simulink subsystem "PvtSubSys_LATC"  (R2020b)
settings: Solver=VariableStepAuto  StartTime=0.0  StopTime=10.0  RelTol=1e-3
undefined symbols (not defined in the file or in its folder): LCS_PLAN_PreViewIdxNum, LCS_PLAN_PreViewIdxSW_b, P_Global_CharSpd_ms, P_Global_SteeringAngleRatio, P_Global_WheelBase_m, P_LCS_DetNoOverRide_DrvTrq_TH, P_LCS_DetOverRide_DrvTrq_TH, P_LCS_ESS_AngleSlope_Limit, P_LCS_ESS_LogicTest_Enable, P_LCS_ESS_NotActiveFlgDelayTime, P_LCS_ESS_NotActiveFlgDelayTimeSW, P_LCS_ESS_SteerAngleErr, P_LCS_ESS_SteerAngleFilterTime, P_LCS_ESS_TarAngleFilterTime, P_LCS_ESSAngleSW, P_LCS_ESSOverrideTime1, P_LCS_ESSOverrideTime2, P_LCS_ESSOverrideTime3, P_LCS_ESSOverrideValue1, P_LCS_ESSOverrideValue2, P_LCS_IN_Offset_Test_SW, P_LCS_IN_Offset_Test_Value, P_LCS_LATC_AngleFilterTime_s, P_LCS_LATC_CurOffsetA2FliterT_s, P_LCS_LATC_CurOffsetCurve_TabX_m, P_LCS_LATC_CurOffsetCurveFliterTime_Tab_s, P_LCS_LATC_CurOffsetVehicleSpdLimitValue_degs, P_LCS_LATC_DeltaEps_Tab_s, P_LCS_LATC_DxOffset_Sw, P_LCS_LATC_ELKAngleSlope_ratio, P_LCS_LATC_ELKMaxLatAcc_ms2, P_LCS_LATC_ESSA0Dis_TabX_m, P_LCS_LATC_ESSAddAngleSlope_Tab_degs, P_LCS_LATC_ESSAESAngleSlope_Tab_degs, P_LCS_LATC_ESSAngleSlope_ratio, P_LCS_LATC_ESSMaxLatAcc_ms2, P_LCS_LATC_LCAngleSlope_ratio, P_LCS_LATC_LCAngleSlope_Tab_degs, P_LCS_LATC_LCCancleMaxLatAcc_ms2, P_LCS_LATC_LCEcoAngleSlope_ratio, P_LCS_LATC_LCEcoAngleSlope_Tab_degs, P_LCS_LATC_LCEcoMaxLatAcc_ms2, P_LCS_LATC_LCKAngleSlope_ratio, P_LCS_LATC_LCKAngleSlope_Tab_degs, P_LCS_LATC_LCKIEAngleSlope_ratio, P_LCS_LATC_LCKIEAngleSlope_Tab_degs, P_LCS_LATC_LCKIEMaxLatAcc_ms2, P_LCS_LATC_LCKMaxLatAcc_ms2, P_LCS_LATC_LCNormalAngleSlope_ratio, P_LCS_LATC_LCNormalAngleSlope_Tab_degs, P_LCS_LATC_LCNormalMaxLatAcc_ms2, P_LCS_LATC_LCSportAngleSlope_ratio, P_LCS_LATC_LCSportAngleSlope_Tab_degs, P_LCS_LATC_LCSportMaxLatAcc_ms2, P_LCS_LATC_LKAAngleSlope_ratio, P_LCS_LATC_LKAAngleSlope_Tab_degs, P_LCS_LATC_LKAMaxLatAcc_ms2, P_LCS_LATC_MatrixQ1_st, P_LCS_LATC_MatrixQ3_st, P_LCS_LATC_MatrixR_st ... (+71)
libraries: simulink x38
(part 3 of 6)

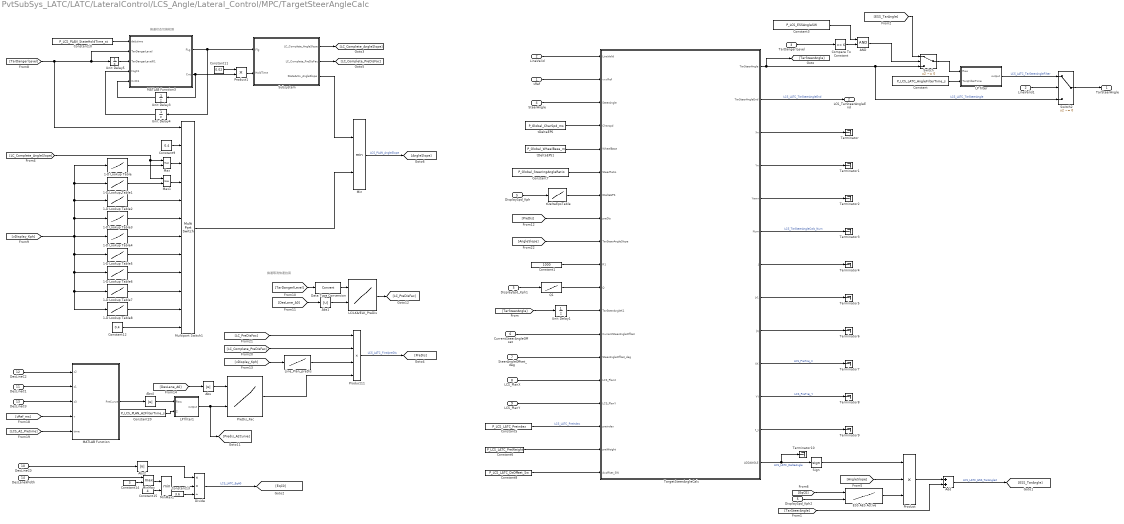
== system PvtSubSys_LATC/LATC/LateralControl/LCS_Angle/Lateral_Control/MPC/TargetSteerAngleCalc ==
  note: 换道状态切换检测
  note: 换道取消快速拉回
  vRef : Inport
  LineValid : Inport  Port=2
  TarDangerlLevel : Inport  Port=3
  SteerAngle : Inport  Port=4
  DisplaySpd_Kph : Inport  Port=5
  CurrentSteerAngleOffset : Inport  Port=6
  SteerAngleOffset_deg : Inport  Port=7
  LCS_PlanX : Inport  Port=8
  LCS_PlanY : Inport  Port=9
  DesLineC0 : Inport  Port=10
  DesLineC1 : Inport  Port=11
  DesLineC2 : Inport  Port=12
  DesLineC3 : Inport  Port=13
  DesLaneWidth : Inport  Port=14
  1-D Lookup Table : Lookup_n-D  NumberOfTableDimensions=1  BreakpointsForDimension1=P_LCS_LATC_VehicleSpd_TabX_Kph  Table=P_LCS_LATC_LCKAngleSlope_Tab_degs  InternalRulePriority=Speed  RndMeth=Simplest  InputSameDT=on
  1-D Lookup Table1 : Lookup_n-D  NumberOfTableDimensions=1  BreakpointsForDimension1=P_LCS_LATC_VehicleSpd_TabX_Kph  Table=P_LCS_LATC_LCKIEAngleSlope_Tab_degs  InternalRulePriority=Speed  RndMeth=Simplest  InputSameDT=on
  1-D Lookup Table2 : Lookup_n-D  NumberOfTableDimensions=1  BreakpointsForDimension1=P_LCS_LATC_VehicleSpd_TabX_Kph  Table=P_LCS_LATC_LCNormalAngleSlope_Tab_degs  InternalRulePriority=Speed  RndMeth=Simplest  InputSameDT=on
  1-D Lookup Table3 : Lookup_n-D  NumberOfTableDimensions=1  BreakpointsForDimension1=P_LCS_LATC_VehicleSpd_TabX_Kph  Table=P_LCS_LATC_LKAAngleSlope_Tab_degs  InternalRulePriority=Speed  RndMeth=Simplest  InputSameDT=on
  1-D Lookup Table4 : Lookup_n-D  NumberOfTableDimensions=1  BreakpointsForDimension1=P_LCS_LATC_VehicleSpd_TabX_Kph  Table=P_LCS_PLAN_ELKAngleSlope_Tab_degs  InternalRulePriority=Speed  RndMeth=Simplest  InputSameDT=on
  1-D Lookup Table5 : Lookup_n-D  NumberOfTableDimensions=1  BreakpointsForDimension1=P_LCS_LATC_VehicleSpd_TabX_Kph  Table=P_LCS_LATC_ESSAESAngleSlope_Tab_degs  InternalRulePriority=Speed  RndMeth=Simplest  InputSameDT=on
  1-D Lookup Table6 : Lookup_n-D  NumberOfTableDimensions=1  BreakpointsForDimension1=P_LCS_LATC_VehicleSpd_TabX_Kph  Table=P_LCS_LATC_LCEcoAngleSlope_Tab_degs  InternalRulePriority=Speed  RndMeth=Simplest  InputSameDT=on
  1-D Lookup Table7 : Lookup_n-D  NumberOfTableDimensions=1  BreakpointsForDimension1=P_LCS_LATC_VehicleSpd_TabX_Kph  Table=P_LCS_LATC_LCSportAngleSlope_Tab_degs  InternalRulePriority=Speed  RndMeth=Simplest  InputSameDT=on
  1-D Lookup Table8 : Lookup_n-D  NumberOfTableDimensions=1  BreakpointsForDimension1=P_LCS_LATC_VehicleSpd_TabX_Kph  Table=P_LCS_LATC_LCAngleSlope_Tab_degs  InternalRulePriority=Speed  RndMeth=Simplest  InputSameDT=on
  AND : Logic  AllPortsSameDT=off  OutDataTypeStr=boolean
  Abs{,1..2,4} (4 alike) : Abs
  Add : Sum
  Compare To Constant : simulink/Logic and Bit Operations/Compare To Constant  relop===  const=6  OutDataTypeStr=boolean
  Constant : Constant  Value=P_LCS_LATC_AngleFilterTime_s  OutDataTypeStr=single
  Constant1 : Constant  Value=1000  OutDataTypeStr=single
  Constant10 : Constant  Value=P_LCS_PLAN_StateHoldTime_st  OutDataTypeStr=uint16
  Constant11 : Constant  Value=0.02
  Constant12 : Constant  Value=0.4  OutDataTypeStr=single
  Constant13 : Constant  Value=3.6  OutDataTypeStr=single
  Constant14 : Constant  Value=3  OutDataTypeStr=single
  Constant15 : Constant  Value=4  OutDataTypeStr=single
  Constant20 : Constant  Value=P_LCS_PLAN_A2FliterTime_s
  Constant3 : Constant  Value=P_LCS_ESSAngleSW  OutDataTypeStr=boolean
  Constant5 : Constant  Value=P_LCS_LATC_Preindex  OutDataTypeStr=single
  Constant6 : Constant  Value=P_LCS_LATC_PreWeight  OutDataTypeStr=single
  Constant7 : Constant  Value=P_Global_SteeringAngleRatio  OutDataTypeStr=single
  Constant8 : Constant  Value=P_LCS_LATC_DxOffset_Sw
  Constant9 : Constant  Value=0.4  OutDataTypeStr=single
  Data Type Conversion : DataTypeConversion
  DisplaySpd_Kph1 : InportShadow  Port=5
  DisplaySpd_Kph2 : InportShadow  Port=5
  Divide : Product  Inputs=**/
  ESS AES Active : Lookup_n-D  BreakpointsForDimension1=P_LCS_LATC_ESSA0Dis_TabX_m  BreakpointsForDimension2=P_LCS_LATC_VehicleSpd_TabX_Kph  Table=P_LCS_LATC_ESSAddAngleSlope_Tab_degs  ExtrapMethod=Clip  UseLastTableValue=on  InternalRulePriority=Speed  OutDataTypeStr=single  RndMeth=Simplest
      settings: InputPortMap=u0,u1
  LC/LKA/ELK_PreDis : Lookup_n-D  BreakpointsForDimension1=P_LCS_PLAN_TarDangerlLevel_Tabx_st  BreakpointsForDimension2=P_LCS_PLAN_DesLineA0_TabY_m  Table=P_LCS_PLAN_LCPreDisFac_ratio  ExtrapMethod=Clip  UseLastTableValue=on  InternalRulePriority=Speed  RndMeth=Simplest  InputSameDT=on
      settings: InputPortMap=u0,u1
  LP filter : Subsystem
  LP filter1 : Subsystem
  LineValid1 : InportShadow  Port=2
  Line_Plan_preDis : Lookup_n-D  NumberOfTableDimensions=1  BreakpointsForDimension1=P_LCS_PLAN_VehicleSpd_TabX_Kph  Table=P_LCS_PLAN_PreDis_Tab_m  ExtrapMethod=Clip  UseLastTableValue=on  InternalRulePriority=Speed  RndMeth=Simplest  InputSameDT=on
  MATLAB Function : MATLAB Function  TreatAsAtomicUnit=on
  MATLAB Function3 : MATLAB Function  TreatAsAtomicUnit=on
  Max : MinMax  Function=max  Inputs=2
  Max1 : MinMax  Function=max  Inputs=2
  Min : MinMax  Inputs=2
  MinMax : MinMax  Function=max  Inputs=2
  MinMax1 : MinMax  Inputs=2
  Multiport Switch1 : MultiPortSwitch  DataPortOrder=Zero-based contiguous  Inputs=11  zeroidx=on
  PreDis_Fac : Lookup_n-D  BreakpointsForDimension1=P_LCS_PLAN_DesLineA0_TabX_m  BreakpointsForDimension2=P_LCS_PLAN_PreDisCurve_TabY_m  Table=P_LCS_PlLAN_PreDisFac_Tab_ratio  ExtrapMethod=Clip  UseLastTableValue=on  InternalRulePriority=Speed  RndMeth=Simplest  InputSameDT=on
      settings: InputPortMap=u0,u1
  Product : Product  Inputs=3  OutDataTypeStr=single
  Product1 : Product
  Product11 : Product  Inputs=4
  Q1 : Lookup_n-D  NumberOfTableDimensions=1  BreakpointsForDimension1=[0,5,10,15,20,25,30,35,40,60,80,90,100,110,120,140]  Table=[0,0,0,0,0,0,0,0,0,0,0,0,0,0,0,0]  InternalRulePriority=Speed  RndMeth=Simplest  InputSameDT=on
  Sign : Signum
  Subsystem : Subsystem
  Switch : Switch  Criteria=u2 ~= 0
  Switch2 : Switch  Criteria=u2 ~= 0
  TargetSteerAngleCalc : MATLAB Function  TreatAsAtomicUnit=on
  Terminator{,1..10} (11 alike) : Terminator
  Unit Delay{1,3..5} (4 alike) : UnitDelay  SampleTime=-1  HasFrameUpgradeWarning=on
  tDeltaEPS : Constant  Value=P_Global_CharSpd_ms
  tDeltaEPS1 : Constant  Value=P_Global_WheelBase_m
  tDeltaEpsTable : Lookup_n-D  NumberOfTableDimensions=1  BreakpointsForDimension1=P_LCS_PLAN_VehicleSpd_TabX_Kph  Table=P_LCS_LATC_DeltaEps_Tab_s  ExtrapMethod=Clip  InternalRulePriority=Speed  RndMeth=Simplest  InputSameDT=on
  TarSteerAngle : Outport
  LCS_TarSteerAngleEnd : Outport  Port=2
  wires:
  Constant8/1 -> TargetSteerAngleCalc/19(dxoffset_SW)
  Constant6/1 -> TargetSteerAngleCalc/18(preWeight)
  Constant5/1 -> TargetSteerAngleCalc/17(preindex)  "LCS_LATC_PreIndex"
  LCS_PlanY/1 -> TargetSteerAngleCalc/16(LCS_PlanY)
  LCS_PlanX/1 -> TargetSteerAngleCalc/15(LCS_PlanX)
  LineValid1/1 -> Switch2/2
  ESS AES Active/1 -> Product/3
  DisplaySpd_Kph2/1 -> ESS AES Active/2
  [EqC0] -> ESS AES Active/1
  TarDangerlLevel/1 -> Compare To Constant/1
  TargetSteerAngleCalc/13(ADDANGLE) -> Sign/1, Terminator10/1  "LCS_LATC_DeltaAngle"
  Sign/1 -> Product/1
  [AngleSlope] -> Product/2
  Product/1 -> Add/1
  [TarSteerAngle] -> Add/2
  Add/1 -> [ESS_TarAngle]  "LCS_LATC_ESS_TarAngle2"
  TargetSteerAngleCalc/1(TarSteerAngle) -> Switch/3, Switch2/3, [TarSteerAngle]  "LCS_LATC_TarSteerAngle"
  Constant/1 -> LP filter/2(TorqFilterTime)
  LP filter/1(output) -> Switch2/1  "LCS_LATC_TarSteerAngleFilter"
  Switch/1 -> LP filter/1(Raw)
  [ESS_TarAngle] -> Switch/1
  Constant3/1 -> AND/1
  Compare To Constant/1 -> AND/2
  AND/1 -> Switch/2
  Switch2/1 -> TarSteerAngle/1
  TargetSteerAngleCalc/12(t_y) -> Terminator9/1
  TargetSteerAngleCalc/2(TarSteerAngleEnd) -> LCS_TarSteerAngleEnd/1  "LCS_LATC_TarSteerAngleEnd"
  [PreDis] -> TargetSteerAngleCalc/8(preDis)
  [AngleSlope] -> TargetSteerAngleCalc/9(TarSteerAngleSlope)
  SteerAngle/1 -> TargetSteerAngleCalc/3(SteerAngle)
  vRef/1 -> TargetSteerAngleCalc/2(vxvRef)
  TargetSteerAngleCalc/11(YY) -> Terminator8/1  "LCS_PreTraj_Y"
  TargetSteerAngleCalc/10(XX) -> Terminator7/1  "LCS_PreTraj_X"
  Constant1/1 -> TargetSteerAngleCalc/10(R1)
  TargetSteerAngleCalc/9(Jq) -> Terminator6/1
  TargetSteerAngleCalc/8(Jr1) -> Terminator5/1
  TargetSteerAngleCalc/7(J) -> Terminator4/1
  TargetSteerAngleCalc/6(Num) -> Terminator3/1  "LCS_TarSteerAngleCalc_Num"
  TargetSteerAngleCalc/5(Yawn) -> Terminator2/1
  TargetSteerAngleCalc/4(Yn) -> Terminator1/1
  TargetSteerAngleCalc/3(Xn) -> Terminator/1
  Constant7/1 -> TargetSteerAngleCalc/6(SteerRatio)
  tDeltaEpsTable/1 -> TargetSteerAngleCalc/7(tDeltaEPS)
  DisplaySpd_Kph/1 -> tDeltaEpsTable/1
  tDeltaEPS/1 -> TargetSteerAngleCalc/4(Charspd)
  tDeltaEPS1/1 -> TargetSteerAngleCalc/5(WheelBase)
  [TarSteerAngle] -> Unit Delay1/1
  Unit Delay1/1 -> TargetSteerAngleCalc/12(TarSteerAngleK1)
  Q1/1 -> TargetSteerAngleCalc/11(Q)
  DisplaySpd_Kph1/1 -> Q1/1
  CurrentSteerAngleOffset/1 -> TargetSteerAngleCalc/13(CurrentSteerAngleOffset)
  LineValid/1 -> TargetSteerAngleCalc/1(LineValid)
  SteerAngleOffset_deg/1 -> TargetSteerAngleCalc/14(SteerAngleOffset_deg)
  Constant12/1 -> Multiport Switch1/12
  1-D Lookup Table7/1 -> Multiport Switch1/10
  MATLAB Function3/1(FLg) -> Unit Delay4/1, Subsystem/1(Flg)
  MATLAB Function3/2(Cnt) -> Product1/2, Unit Delay3/1
  Unit Delay3/1 -> MATLAB Function3/5(CntK1)
  1-D Lookup Table4/1 -> Multiport Switch1/7
  1-D Lookup Table/1 -> Max/2
  Unit Delay5/1 -> MATLAB Function3/3(TarDangerLevelK1)
  1-D Lookup Table2/1 -> Multiport Switch1/5
  1-D Lookup Table5/1 -> Multiport Switch1/8
  1-D Lookup Table6/1 -> Multiport Switch1/9
  Max1/1 -> Multiport Switch1/4
  Max/1 -> Multiport Switch1/3
  [LC_Complete_AngleSlope] -> Max1/1, Max/1
  [TarDangerlLevel] -> MATLAB Function3/2(TarDangerLevel), Unit Delay5/1, Multiport Switch1/1
  Constant9/1 -> Multiport Switch1/2
  Constant10/1 -> MATLAB Function3/1(delytime)
  1-D Lookup Table3/1 -> Multiport Switch1/6
  Product1/1 -> Subsystem/2(HoldTime)
  1-D Lookup Table8/1 -> Multiport Switch1/11
  Min/1 -> [AngleSlope]  "LCS_PLAN_AngleSlope"
  Unit Delay4/1 -> MATLAB Function3/4(FLgK1)
  Multiport Switch1/1 -> Min/2
  1-D Lookup Table1/1 -> Max1/2
  Constant11/1 -> Product1/1
  PreDis_Fac/1 -> Product11/4
  Line_Plan_preDis/1 -> Product11/3
  MATLAB Function/1(PreCurve) -> Abs4/1
  DesLineC2/1 -> MATLAB Function/1(c2)
  [vRef_ms] -> MATLAB Function/4(v)
  Data Type Conversion/1 -> LC/LKA/ELK_PreDis/1
  Abs/1 -> PreDis_Fac/1
  [DesLane_A0] -> Abs1/1
  Abs1/1 -> LC/LKA/ELK_PreDis/2
  [vDisplay_Kph] -> Line_Plan_preDis/1
  LC/LKA/ELK_PreDis/1 -> [LC_PreDisFac]
  [TarDangerlLevel] -> Data Type Conversion/1
  [DesLane_A0] -> Abs/1
  DesLineC3/1 -> MATLAB Function/3(c3)
  Constant20/1 -> LP filter1/2(TorqFilterTime)
  Abs4/1 -> LP filter1/1(Raw)
  Product11/1 -> [PreDis]  "LCS_LATC_FinalpreDis"
  [LC_PreDisFac] -> Product11/1
  LP filter1/1(output) -> PreDis_Fac/2, [Predis_A2Curve]
  [LC_Complete_PreDisFac] -> Product11/2
  [LCS_A2_Pretime] -> MATLAB Function/5(time)
  DesLineC1/1 -> MATLAB Function/2(c1)
  [vDisplay_Kph] -> 1-D Lookup Table8/1, 1-D Lookup Table7/1, 1-D Lookup Table6/1, 1-D Lookup Table5/1, 1-D Lookup Table2/1, 1-D Lookup Table1/1, 1-D Lookup Table/1, 1-D Lookup Table3/1, 1-D Lookup Table4/1
  Subsystem/1(LC_Complete_AngleSlope) -> [LC_Complete_AngleSlope]
  Subsystem/3(StateActiv_AngleSlope) -> Min/1
  Subsystem/2(LC_Complete_PreDisFac) -> [LC_Complete_PreDisFac]
  Constant15/1 -> MinMax1/2
  Constant13/1 -> Divide/3
  MinMax1/1 -> Divide/2
  DesLineC0/1 -> Abs2/1
  MinMax/1 -> MinMax1/1
  Divide/1 -> [EqC0]  "LCS_LATC_EqA0"
  Constant14/1 -> MinMax/2
  DesLaneWidth/1 -> MinMax/1
  Abs2/1 -> Divide/1

== system PvtSubSys_LATC/LATC/LateralControl/LCS_Angle/Lateral_Control/MPC/Understeer_Offset_Calc ==
  note: %% 匀速
  SteerAngle_deg : Inport
  PsiDtOpt : Inport  Port=2
  axvRef : Inport  Port=3
  DesLineC2 : Inport  Port=4
  vxvRef : Inport  Port=5
  Abs : Abs
  Abs2 : Abs
  Compare To Constant1 : simulink/Logic and Bit Operations/Compare To Constant  relop=>  const=P_LCS_LATC_CurOffsetVehicleSpdLimitValue_degs  OutDataTypeStr=boolean
  Compare To Constant6 : simulink/Logic and Bit Operations/Compare To Constant  relop=<=  const=1.5  OutDataTypeStr=boolean
  Constant1 : Constant  Value=P_Global_SteeringAngleRatio
  Constant2 : Constant  Value=P_LCS_LATC_CurOffsetA2FliterT_s  OutDataTypeStr=single
  Constant4 : Constant  Value=P_Global_CharSpd_ms
  Constant5 : Constant  Value=P_Global_WheelBase_m
  Constant6 : Constant  Value=57.3  OutDataTypeStr=single
  Enabled Subsystem : Subsystem  TreatAsAtomicUnit=on
  FilterTime2 : Product  Inputs=*//  RndMeth=Zero
  Gain : Gain  Gain=2
  LP filter : Subsystem
  Logical Operator : Logic  AllPortsSameDT=off  OutDataTypeStr=boolean
  Memory52 : Memory  InheritSampleTime=on
  Sum : Sum  Inputs=+-
  Terminator : Terminator
  YOD_Ackman : MATLAB Function  TreatAsAtomicUnit=on
  SteerAngleOffset_deg : Outport
  wires:
  Constant2/1 -> LP filter/2(TorqFilterTime)
  DesLineC2/1 -> Gain/1
  Gain/1 -> Abs/1
  Abs/1 -> LP filter/1(Raw)
  SteerAngle_deg/1 -> FilterTime2/1
  Compare To Constant1/1 -> Logical Operator/2
  YOD_Ackman/2(PsiDtAck) -> Memory52/1, Sum/1
  Enabled Subsystem/1(SteerAngleOffset_deg) -> SteerAngleOffset_deg/1
  Constant5/1 -> YOD_Ackman/3(WheelBase)
  Constant4/1 -> YOD_Ackman/2(Vch)
  Memory52/1 -> YOD_Ackman/5(PsiDtAckK1)
  PsiDtOpt/1 -> Sum/2
  vxvRef/1 -> YOD_Ackman/1(VxvRef), Compare To Constant1/1
  Sum/1 -> Enabled Subsystem/2(Raw)
  Logical Operator/1 -> Enabled Subsystem/Enable, Terminator/1  "LCS_OffSetUpdate_Flg"
  Constant1/1 -> FilterTime2/2
  Constant6/1 -> FilterTime2/3
  YOD_Ackman/1(AckConst) -> Enabled Subsystem/1(AckConst)
  FilterTime2/1 -> YOD_Ackman/4(AlpWheelAngle)
  axvRef/1 -> Abs2/1
  Abs2/1 -> Compare To Constant6/1
  Compare To Constant6/1 -> Logical Operator/1
  LP filter/1(output) -> Enabled Subsystem/3(Curve)

== system PvtSubSys_LATC/LATC/LateralControl/LCS_Angle/Lateral_Control/Trajectory_MPC/Median_Filter ==
  In : Inport
  Constant11 : Constant  Value=P_LCS_LCC_TarAngleFliterWindowSize - single(2)  OutDataTypeStr=single
  Divide1 : Product  Inputs=*/
  Max of Elements1 : MinMax  Function=max
  MinMax2 : MinMax
  Minus1 : Sum  Inputs=--+
  Sum of Elements1 : Sum  Inputs=+
  Tapped Delay1 : simulink/Discrete/Tapped Delay  vinit=0.0  samptime=-1  NumDelays=P_LCS_LCC_TarAngleFliterWindowSize-1  DelayOrder=Newest  includeCurrent=on
  Out : Outport
  wires:
  Max of Elements1/1 -> Minus1/2
  Divide1/1 -> Out/1
  Minus1/1 -> Divide1/1
  In/1 -> Tapped Delay1/1
  MinMax2/1 -> Minus1/1
  Sum of Elements1/1 -> Minus1/3
  Tapped Delay1/1 -> Max of Elements1/1, MinMax2/1, Sum of Elements1/1
  Constant11/1 -> Divide1/2

== system PvtSubSys_LATC/LATC/LateralControl/LCS_Angle/Lateral_Control/Trajectory_MPC/Subsystem5 ==
  raw : Inport
  Slope : Inport  Port=2
  Add : Sum
  Add1 : Sum  Inputs=+-
  Max : MinMax  Inputs=2
  Min : MinMax  Function=max  Inputs=2
  Unit Delay : UnitDelay  InitialCondition=single(0)  SampleTime=-1  HasFrameUpgradeWarning=on
  out : Outport
  wires:
  raw/1 -> Max/2
  Add1/1 -> Min/2
  Add/1 -> Max/1
  Max/1 -> Min/1
  Min/1 -> Unit Delay/1, out/1
  Unit Delay/1 -> Add/1, Add1/1
  Slope/1 -> Add/2, Add1/2

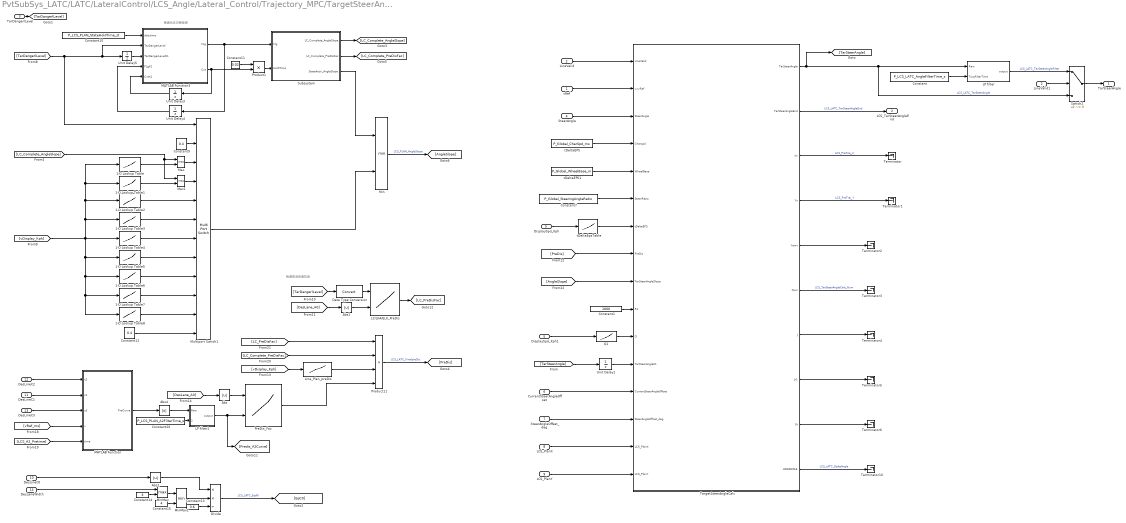
== system PvtSubSys_LATC/LATC/LateralControl/LCS_Angle/Lateral_Control/Trajectory_MPC/TargetSteerAngleCalc ==
  note: 换道取消快速拉回
  note: 换道状态切换检测
  vRef : Inport
  LineValid : Inport  Port=2
  TarDangerlLevel : Inport  Port=3
  SteerAngle : Inport  Port=4
  DisplaySpd_Kph : Inport  Port=5
  CurrentSteerAngleOffset : Inport  Port=6
  SteerAngleOffset_deg : Inport  Port=7
  LCS_PlanX : Inport  Port=8
  LCS_PlanY : Inport  Port=9
  DesLineC0 : Inport  Port=10
  DesLineC1 : Inport  Port=11
  DesLineC2 : Inport  Port=12
  DesLineC3 : Inport  Port=13
  DesLaneWidth : Inport  Port=14
  1-D Lookup Table : Lookup_n-D  NumberOfTableDimensions=1  BreakpointsForDimension1=P_LCS_LATC_VehicleSpd_TabX_Kph  Table=P_LCS_LATC_LCKAngleSlope_Tab_degs  InternalRulePriority=Speed  RndMeth=Simplest  InputSameDT=on
  1-D Lookup Table1 : Lookup_n-D  NumberOfTableDimensions=1  BreakpointsForDimension1=P_LCS_LATC_VehicleSpd_TabX_Kph  Table=P_LCS_LATC_LCKIEAngleSlope_Tab_degs  InternalRulePriority=Speed  RndMeth=Simplest  InputSameDT=on
  1-D Lookup Table2 : Lookup_n-D  NumberOfTableDimensions=1  BreakpointsForDimension1=P_LCS_LATC_VehicleSpd_TabX_Kph  Table=P_LCS_LATC_LCNormalAngleSlope_Tab_degs  InternalRulePriority=Speed  RndMeth=Simplest  InputSameDT=on
  1-D Lookup Table3 : Lookup_n-D  NumberOfTableDimensions=1  BreakpointsForDimension1=P_LCS_LATC_VehicleSpd_TabX_Kph  Table=P_LCS_LATC_LKAAngleSlope_Tab_degs  InternalRulePriority=Speed  RndMeth=Simplest  InputSameDT=on
  1-D Lookup Table4 : Lookup_n-D  NumberOfTableDimensions=1  BreakpointsForDimension1=P_LCS_LATC_VehicleSpd_TabX_Kph  Table=P_LCS_PLAN_ELKAngleSlope_Tab_degs  InternalRulePriority=Speed  RndMeth=Simplest  InputSameDT=on
  1-D Lookup Table5 : Lookup_n-D  NumberOfTableDimensions=1  BreakpointsForDimension1=P_LCS_LATC_VehicleSpd_TabX_Kph  Table=P_LCS_LATC_ESSAESAngleSlope_Tab_degs  InternalRulePriority=Speed  RndMeth=Simplest  InputSameDT=on
  1-D Lookup Table6 : Lookup_n-D  NumberOfTableDimensions=1  BreakpointsForDimension1=P_LCS_LATC_VehicleSpd_TabX_Kph  Table=P_LCS_LATC_LCEcoAngleSlope_Tab_degs  InternalRulePriority=Speed  RndMeth=Simplest  InputSameDT=on
  1-D Lookup Table7 : Lookup_n-D  NumberOfTableDimensions=1  BreakpointsForDimension1=P_LCS_LATC_VehicleSpd_TabX_Kph  Table=P_LCS_LATC_LCSportAngleSlope_Tab_degs  InternalRulePriority=Speed  RndMeth=Simplest  InputSameDT=on
  1-D Lookup Table8 : Lookup_n-D  NumberOfTableDimensions=1  BreakpointsForDimension1=P_LCS_LATC_VehicleSpd_TabX_Kph  Table=P_LCS_LATC_LCAngleSlope_Tab_degs  InternalRulePriority=Speed  RndMeth=Simplest  InputSameDT=on
  Abs{,1..2,4} (4 alike) : Abs
  Constant : Constant  Value=P_LCS_LATC_AngleFilterTime_s  OutDataTypeStr=single
  Constant1 : Constant  Value=1000  OutDataTypeStr=single
  Constant10 : Constant  Value=P_LCS_PLAN_StateHoldTime_st  OutDataTypeStr=uint16
  Constant11 : Constant  Value=0.02
  Constant12 : Constant  Value=0.4  OutDataTypeStr=single
  Constant13 : Constant  Value=3.6  OutDataTypeStr=single
  Constant14 : Constant  Value=3  OutDataTypeStr=single
  Constant15 : Constant  Value=4  OutDataTypeStr=single
  Constant20 : Constant  Value=P_LCS_PLAN_A2FliterTime_s
  Constant7 : Constant  Value=P_Global_SteeringAngleRatio  OutDataTypeStr=single
  Constant9 : Constant  Value=0.4  OutDataTypeStr=single
  Data Type Conversion : DataTypeConversion
  DisplaySpd_Kph1 : InportShadow  Port=5
  Divide : Product  Inputs=**/
  LC/LKA/ELK_PreDis : Lookup_n-D  BreakpointsForDimension1=P_LCS_PLAN_TarDangerlLevel_Tabx_st  BreakpointsForDimension2=P_LCS_PLAN_DesLineA0_TabY_m  Table=P_LCS_PLAN_LCPreDisFac_ratio  ExtrapMethod=Clip  UseLastTableValue=on  InternalRulePriority=Speed  RndMeth=Simplest  InputSameDT=on
      settings: InputPortMap=u0,u1
  LP filter : Subsystem
  LP filter1 : Subsystem
  LineValid1 : InportShadow  Port=2
  Line_Plan_preDis : Lookup_n-D  NumberOfTableDimensions=1  BreakpointsForDimension1=P_LCS_PLAN_VehicleSpd_TabX_Kph  Table=P_LCS_PLAN_PreDis_Tab_m  ExtrapMethod=Clip  UseLastTableValue=on  InternalRulePriority=Speed  RndMeth=Simplest  InputSameDT=on
  MATLAB Function : MATLAB Function  TreatAsAtomicUnit=on
  MATLAB Function3 : MATLAB Function  TreatAsAtomicUnit=on
  Max : MinMax  Function=max  Inputs=2
  Max1 : MinMax  Function=max  Inputs=2
  Min : MinMax  Inputs=2
  MinMax : MinMax  Function=max  Inputs=2
  MinMax1 : MinMax  Inputs=2
  Multiport Switch1 : MultiPortSwitch  DataPortOrder=Zero-based contiguous  Inputs=11  zeroidx=on
  PreDis_Fac : Lookup_n-D  BreakpointsForDimension1=P_LCS_PLAN_DesLineA0_TabX_m  BreakpointsForDimension2=P_LCS_PLAN_PreDisCurve_TabY_m  Table=P_LCS_PlLAN_PreDisFac_Tab_ratio  ExtrapMethod=Clip  UseLastTableValue=on  InternalRulePriority=Speed  RndMeth=Simplest  InputSameDT=on
      settings: InputPortMap=u0,u1
  Product1 : Product
  Product11 : Product  Inputs=4
  Q1 : Lookup_n-D  NumberOfTableDimensions=1  BreakpointsForDimension1=[0,5,10,15,20,25,30,35,40,60,80,90,100,110,120,140]  Table=[0,0,0,0,0,0,0,0,0,0,0,0,0,0,0,0]  InternalRulePriority=Speed  RndMeth=Simplest  InputSameDT=on
  Subsystem : Subsystem
  Switch2 : Switch  Criteria=u2 ~= 0
  TargetSteerAngleCalc : MATLAB Function  TreatAsAtomicUnit=on
  Terminator{,1..6,10} (8 alike) : Terminator
  Unit Delay{1,3..5} (4 alike) : UnitDelay  SampleTime=-1  HasFrameUpgradeWarning=on
  tDeltaEPS : Constant  Value=P_Global_CharSpd_ms
  tDeltaEPS1 : Constant  Value=P_Global_WheelBase_m
  tDeltaEpsTable : Lookup_n-D  NumberOfTableDimensions=1  BreakpointsForDimension1=P_LCS_PLAN_VehicleSpd_TabX_Kph  Table=P_LCS_LATC_DeltaEps_Tab_s  ExtrapMethod=Clip  InternalRulePriority=Speed  RndMeth=Simplest  InputSameDT=on
  TarSteerAngle : Outport
  LCS_TarSteerAngleEnd : Outport  Port=2
  wires:
  TarDangerlLevel/1 -> [TarDangerlLevel]
  Abs2/1 -> Divide/1
  DesLaneWidth/1 -> MinMax/1
  Constant14/1 -> MinMax/2
  Divide/1 -> [EqC0]  "LCS_LATC_EqA0"
  MinMax/1 -> MinMax1/1
  DesLineC0/1 -> Abs2/1
  MinMax1/1 -> Divide/2
  Constant13/1 -> Divide/3
  Constant15/1 -> MinMax1/2
  Subsystem/2(LC_Complete_PreDisFac) -> [LC_Complete_PreDisFac]
  Subsystem/3(StateActiv_AngleSlope) -> Min/1
  Subsystem/1(LC_Complete_AngleSlope) -> [LC_Complete_AngleSlope]
  [vDisplay_Kph] -> 1-D Lookup Table4/1, 1-D Lookup Table3/1, 1-D Lookup Table/1, 1-D Lookup Table1/1, 1-D Lookup Table2/1, 1-D Lookup Table5/1, 1-D Lookup Table6/1, 1-D Lookup Table7/1, 1-D Lookup Table8/1
  DesLineC1/1 -> MATLAB Function/2(c1)
  [LCS_A2_Pretime] -> MATLAB Function/5(time)
  [LC_Complete_PreDisFac] -> Product11/2
  LP filter1/1(output) -> [Predis_A2Curve], PreDis_Fac/2
  [LC_PreDisFac] -> Product11/1
  Product11/1 -> [PreDis]  "LCS_LATC_FinalpreDis"
  Abs4/1 -> LP filter1/1(Raw)
  Constant20/1 -> LP filter1/2(TorqFilterTime)
  DesLineC3/1 -> MATLAB Function/3(c3)
  [DesLane_A0] -> Abs/1
  [TarDangerlLevel] -> Data Type Conversion/1
  LC/LKA/ELK_PreDis/1 -> [LC_PreDisFac]
  [vDisplay_Kph] -> Line_Plan_preDis/1
  Abs1/1 -> LC/LKA/ELK_PreDis/2
  [DesLane_A0] -> Abs1/1
  Abs/1 -> PreDis_Fac/1
  Data Type Conversion/1 -> LC/LKA/ELK_PreDis/1
  [vRef_ms] -> MATLAB Function/4(v)
  DesLineC2/1 -> MATLAB Function/1(c2)
  MATLAB Function/1(PreCurve) -> Abs4/1
  Line_Plan_preDis/1 -> Product11/3
  PreDis_Fac/1 -> Product11/4
  Constant11/1 -> Product1/1
  1-D Lookup Table1/1 -> Max1/2
  Multiport Switch1/1 -> Min/2
  Unit Delay4/1 -> MATLAB Function3/4(FLgK1)
  Min/1 -> [AngleSlope]  "LCS_PLAN_AngleSlope"
  1-D Lookup Table8/1 -> Multiport Switch1/11
  Product1/1 -> Subsystem/2(HoldTime)
  1-D Lookup Table3/1 -> Multiport Switch1/6
  Constant10/1 -> MATLAB Function3/1(delytime)
  Constant9/1 -> Multiport Switch1/2
  [TarDangerlLevel] -> Multiport Switch1/1, Unit Delay5/1, MATLAB Function3/2(TarDangerLevel)
  [LC_Complete_AngleSlope] -> Max/1, Max1/1
  Max/1 -> Multiport Switch1/3
  Max1/1 -> Multiport Switch1/4
  1-D Lookup Table6/1 -> Multiport Switch1/9
  1-D Lookup Table5/1 -> Multiport Switch1/8
  1-D Lookup Table2/1 -> Multiport Switch1/5
  Unit Delay5/1 -> MATLAB Function3/3(TarDangerLevelK1)
  1-D Lookup Table/1 -> Max/2
  1-D Lookup Table4/1 -> Multiport Switch1/7
  Unit Delay3/1 -> MATLAB Function3/5(CntK1)
  MATLAB Function3/2(Cnt) -> Unit Delay3/1, Product1/2
  MATLAB Function3/1(FLg) -> Subsystem/1(Flg), Unit Delay4/1
  1-D Lookup Table7/1 -> Multiport Switch1/10
  Constant12/1 -> Multiport Switch1/12
  SteerAngleOffset_deg/1 -> TargetSteerAngleCalc/14(SteerAngleOffset_deg)
  LineValid/1 -> TargetSteerAngleCalc/1(LineValid)
  CurrentSteerAngleOffset/1 -> TargetSteerAngleCalc/13(CurrentSteerAngleOffset)
  DisplaySpd_Kph1/1 -> Q1/1
  Q1/1 -> TargetSteerAngleCalc/11(Q)
  Unit Delay1/1 -> TargetSteerAngleCalc/12(TarSteerAngleK1)
  [TarSteerAngle] -> Unit Delay1/1
  tDeltaEPS1/1 -> TargetSteerAngleCalc/5(WheelBase)
  tDeltaEPS/1 -> TargetSteerAngleCalc/4(Charspd)
  DisplaySpd_Kph/1 -> tDeltaEpsTable/1
  tDeltaEpsTable/1 -> TargetSteerAngleCalc/7(tDeltaEPS)
  Constant7/1 -> TargetSteerAngleCalc/6(SteerRatio)
  TargetSteerAngleCalc/3(Xn) -> Terminator/1  "LCS_PreTraj_X"
  TargetSteerAngleCalc/4(Yn) -> Terminator1/1  "LCS_PreTraj_Y"
  TargetSteerAngleCalc/5(Yawn) -> Terminator2/1
  TargetSteerAngleCalc/6(Num) -> Terminator3/1  "LCS_TarSteerAngleCalc_Num"
  TargetSteerAngleCalc/7(J) -> Terminator4/1
  TargetSteerAngleCalc/8(Jr1) -> Terminator5/1
  TargetSteerAngleCalc/9(Jq) -> Terminator6/1
  Constant1/1 -> TargetSteerAngleCalc/10(R1)
  vRef/1 -> TargetSteerAngleCalc/2(vxvRef)
  SteerAngle/1 -> TargetSteerAngleCalc/3(SteerAngle)
  [AngleSlope] -> TargetSteerAngleCalc/9(TarSteerAngleSlope)
  [PreDis] -> TargetSteerAngleCalc/8(PreDis)
  TargetSteerAngleCalc/2(TarSteerAngleEnd) -> LCS_TarSteerAngleEnd/1  "LCS_LATC_TarSteerAngleEnd"
  Switch2/1 -> TarSteerAngle/1
  LP filter/1(output) -> Switch2/1  "LCS_LATC_TarSteerAngleFilter"
  Constant/1 -> LP filter/2(TorqFilterTime)
  TargetSteerAngleCalc/1(TarSteerAngle) -> LP filter/1(Raw), Switch2/3, [TarSteerAngle]  "LCS_LATC_TarSteerAngle"
  TargetSteerAngleCalc/10(ADDANGLE) -> Terminator10/1  "LCS_LATC_DeltaAngle"
  LineValid1/1 -> Switch2/2
  LCS_PlanX/1 -> TargetSteerAngleCalc/15(LCS_PlanX)
  LCS_PlanY/1 -> TargetSteerAngleCalc/16(LCS_PlanY)

== system PvtSubSys_LATC/LATC/LateralControl/LCS_Angle/Lateral_Control/Trajectory_MPC/Understeer_Offset_Calc ==
  note: %% 匀速
  SteerAngle_deg : Inport
  PsiDtOpt : Inport  Port=2
  axvRef : Inport  Port=3
  DesLineC2 : Inport  Port=4
  vxvRef : Inport  Port=5
  Abs : Abs
  Abs2 : Abs
  Compare To Constant1 : simulink/Logic and Bit Operations/Compare To Constant  relop=>  const=P_LCS_LATC_CurOffsetVehicleSpdLimitValue_degs  OutDataTypeStr=boolean
  Compare To Constant6 : simulink/Logic and Bit Operations/Compare To Constant  relop=<=  const=1.5  OutDataTypeStr=boolean
  Constant1 : Constant  Value=P_Global_SteeringAngleRatio
  Constant2 : Constant  Value=P_LCS_LATC_CurOffsetA2FliterT_s  OutDataTypeStr=single
  Constant4 : Constant  Value=P_Global_CharSpd_ms
  Constant5 : Constant  Value=P_Global_WheelBase_m
  Constant6 : Constant  Value=57.3  OutDataTypeStr=single
  Enabled Subsystem : Subsystem  TreatAsAtomicUnit=on
  FilterTime2 : Product  Inputs=*//  RndMeth=Zero
  Gain : Gain  Gain=2
  LP filter : Subsystem
  Logical Operator : Logic  AllPortsSameDT=off  OutDataTypeStr=boolean
  Memory52 : Memory  InheritSampleTime=on
  Sum : Sum  Inputs=+-
  Terminator : Terminator
  YOD_Ackman : MATLAB Function  TreatAsAtomicUnit=on
  SteerAngleOffset_deg : Outport
  wires:
  LP filter/1(output) -> Enabled Subsystem/3(Curve)
  Compare To Constant6/1 -> Logical Operator/1
  Abs2/1 -> Compare To Constant6/1
  axvRef/1 -> Abs2/1
  FilterTime2/1 -> YOD_Ackman/4(AlpWheelAngle)
  YOD_Ackman/1(AckConst) -> Enabled Subsystem/1(AckConst)
  Constant6/1 -> FilterTime2/3
  Constant1/1 -> FilterTime2/2
  Logical Operator/1 -> Terminator/1, Enabled Subsystem/Enable  "LCS_OffSetUpdate_Flg"
  Sum/1 -> Enabled Subsystem/2(Raw)
  vxvRef/1 -> Compare To Constant1/1, YOD_Ackman/1(VxvRef)
  PsiDtOpt/1 -> Sum/2
  Memory52/1 -> YOD_Ackman/5(PsiDtAckK1)
  Constant4/1 -> YOD_Ackman/2(Vch)
  Constant5/1 -> YOD_Ackman/3(WheelBase)
  Enabled Subsystem/1(SteerAngleOffset_deg) -> SteerAngleOffset_deg/1
  YOD_Ackman/2(PsiDtAck) -> Sum/1, Memory52/1
  Compare To Constant1/1 -> Logical Operator/2
  SteerAngle_deg/1 -> FilterTime2/1
  Abs/1 -> LP filter/1(Raw)
  Gain/1 -> Abs/1
  DesLineC2/1 -> Gain/1
  Constant2/1 -> LP filter/2(TorqFilterTime)

== system PvtSubSys_LATC/LATC/LateralControl/LCS_Angle/Lateral_Control/kinematics_MPC/Median_Filter ==
  In : Inport
  Constant11 : Constant  Value=P_LCS_LATC_TarAngleFliterWindowSize - single(2)  OutDataTypeStr=single
  Divide1 : Product  Inputs=*/
  Max of Elements1 : MinMax  Function=max
  MinMax2 : MinMax
  Minus1 : Sum  Inputs=--+
  Sum of Elements1 : Sum  Inputs=+
  Tapped Delay1 : simulink/Discrete/Tapped Delay  vinit=0.0  samptime=-1  NumDelays=P_LCS_LATC_TarAngleFliterWindowSize-1  DelayOrder=Newest  includeCurrent=on
  Out : Outport
  wires:
  Max of Elements1/1 -> Minus1/2
  Divide1/1 -> Out/1
  Minus1/1 -> Divide1/1
  In/1 -> Tapped Delay1/1
  MinMax2/1 -> Minus1/1
  Sum of Elements1/1 -> Minus1/3
  Tapped Delay1/1 -> Max of Elements1/1, MinMax2/1, Sum of Elements1/1
  Constant11/1 -> Divide1/2

== system PvtSubSys_LATC/LATC/LateralControl/LCS_Angle/Lateral_Control/kinematics_MPC/SteerAngSlopeCalc ==
  note: 换道状态切换检测
  note: 0:No Function Active
      | 1:LCK Active
      | 2:LCKIE Active
      | 3:LC Normal Active
      | 4:LKA Active
      | 5:ELK Active
      | 6:ESS AES Active
      | 7:LC Eco Active
      | 8:LC Sport Active
      | 9:LC cancel
  TarDangerlLevel : Inport
  VehSpd_kph : Inport  Port=2
  Constant : Constant  Value=0.4  OutDataTypeStr=single
  Constant1 : Constant  Value=1.5  OutDataTypeStr=single
  Constant2 : Constant  Value=P_LCS_LATC_StateHoldTime_st  OutDataTypeStr=uint16
  Constant3 : Constant  Value=0.02
  Constant4 : Constant  Value=0.4  OutDataTypeStr=single
  Constant5 : Constant  Value=1.5  OutDataTypeStr=single
  Data Type Conversion : DataTypeConversion  OutDataTypeStr=single
  Data Type Conversion1 : DataTypeConversion  OutDataTypeStr=single
  ELK Active : Lookup_n-D  NumberOfTableDimensions=1  BreakpointsForDimension1=P_LCS_VehicleSpd_TabX_Kph  Table=P_LCS_LATC_ELKAngleSlope_ratio  ExtrapMethod=Clip  InternalRulePriority=Speed  RndMeth=Simplest  InputSameDT=on
  ELK_MaxAy : Lookup_n-D  NumberOfTableDimensions=1  BreakpointsForDimension1=P_LCS_VehicleSpd_TabX_Kph  Table=P_LCS_LATC_ELKMaxLatAcc_ms2  ExtrapMethod=Clip  InternalRulePriority=Speed  RndMeth=Simplest  InputSameDT=on
  ESS AES Active : Lookup_n-D  NumberOfTableDimensions=1  BreakpointsForDimension1=P_LCS_VehicleSpd_TabX_Kph  Table=P_LCS_LATC_ESSAngleSlope_ratio  ExtrapMethod=Clip  InternalRulePriority=Speed  RndMeth=Simplest  InputSameDT=on
  ESS AES_MaxAy : Lookup_n-D  NumberOfTableDimensions=1  BreakpointsForDimension1=P_LCS_VehicleSpd_TabX_Kph  Table=P_LCS_LATC_ESSMaxLatAcc_ms2  ExtrapMethod=Clip  InternalRulePriority=Speed  RndMeth=Simplest  InputSameDT=on
  LC Cancel : Lookup_n-D  NumberOfTableDimensions=1  BreakpointsForDimension1=P_LCS_VehicleSpd_TabX_Kph  Table=P_LCS_LATC_LCAngleSlope_ratio  ExtrapMethod=Clip  InternalRulePriority=Speed  RndMeth=Simplest  InputSameDT=on
  LCK/IE TO LC_Eco : Lookup_n-D  NumberOfTableDimensions=1  BreakpointsForDimension1=P_LCS_VehicleSpd_TabX_Kph  Table=P_LCS_LATC_LCEcoAngleSlope_ratio  ExtrapMethod=Clip  InternalRulePriority=Speed  RndMeth=Simplest  InputSameDT=on
  LCK/IE TO LC_Nomal : Lookup_n-D  NumberOfTableDimensions=1  BreakpointsForDimension1=P_LCS_VehicleSpd_TabX_Kph  Table=P_LCS_LATC_LCNormalAngleSlope_ratio  ExtrapMethod=Clip  InternalRulePriority=Speed  RndMeth=Simplest  InputSameDT=on
  LCK/IE TO LC_Sport : Lookup_n-D  NumberOfTableDimensions=1  BreakpointsForDimension1=P_LCS_VehicleSpd_TabX_Kph  Table=P_LCS_LATC_LCSportAngleSlope_ratio  ExtrapMethod=Clip  InternalRulePriority=Speed  RndMeth=Simplest  InputSameDT=on
  LCKIEMaxAy : Lookup_n-D  NumberOfTableDimensions=1  BreakpointsForDimension1=P_LCS_VehicleSpd_TabX_Kph  Table=P_LCS_LATC_LCKIEMaxLatAcc_ms2  ExtrapMethod=Clip  InternalRulePriority=Speed  RndMeth=Simplest  InputSameDT=on
  LCKIE_Active : Lookup_n-D  NumberOfTableDimensions=1  BreakpointsForDimension1=P_LCS_VehicleSpd_TabX_Kph  Table=P_LCS_LATC_LCKIEAngleSlope_ratio  ExtrapMethod=Clip  InternalRulePriority=Speed  RndMeth=Simplest  InputSameDT=on
  LCKMaxAy : Lookup_n-D  NumberOfTableDimensions=1  BreakpointsForDimension1=P_LCS_VehicleSpd_TabX_Kph  Table=P_LCS_LATC_LCKMaxLatAcc_ms2  ExtrapMethod=Clip  InternalRulePriority=Speed  RndMeth=Simplest  InputSameDT=on
  LCNomal_MaxAy : Lookup_n-D  NumberOfTableDimensions=1  BreakpointsForDimension1=P_LCS_VehicleSpd_TabX_Kph  Table=P_LCS_LATC_LCNormalMaxLatAcc_ms2  ExtrapMethod=Clip  InternalRulePriority=Speed  RndMeth=Simplest  InputSameDT=on
  LC_CancelMaxAy : Lookup_n-D  NumberOfTableDimensions=1  BreakpointsForDimension1=P_LCS_VehicleSpd_TabX_Kph  Table=P_LCS_LATC_LCCancleMaxLatAcc_ms2  ExtrapMethod=Clip  InternalRulePriority=Speed  RndMeth=Simplest  InputSameDT=on
  LC_Eco_MaxAy : Lookup_n-D  NumberOfTableDimensions=1  BreakpointsForDimension1=P_LCS_VehicleSpd_TabX_Kph  Table=P_LCS_LATC_LCEcoMaxLatAcc_ms2  ExtrapMethod=Clip  InternalRulePriority=Speed  RndMeth=Simplest  InputSameDT=on
  LC_SportMaxAy : Lookup_n-D  NumberOfTableDimensions=1  BreakpointsForDimension1=P_LCS_VehicleSpd_TabX_Kph  Table=P_LCS_LATC_LCSportMaxLatAcc_ms2  ExtrapMethod=Clip  InternalRulePriority=Speed  RndMeth=Simplest  InputSameDT=on
  LKA Active : Lookup_n-D  NumberOfTableDimensions=1  BreakpointsForDimension1=P_LCS_VehicleSpd_TabX_Kph  Table=P_LCS_LATC_LKAAngleSlope_ratio  ExtrapMethod=Clip  InternalRulePriority=Speed  RndMeth=Simplest  InputSameDT=on
  LKA_MaxAy : Lookup_n-D  NumberOfTableDimensions=1  BreakpointsForDimension1=P_LCS_VehicleSpd_TabX_Kph  Table=P_LCS_LATC_LKAMaxLatAcc_ms2  ExtrapMethod=Clip  InternalRulePriority=Speed  RndMeth=Simplest  InputSameDT=on
  MATLAB Function3 : MATLAB Function  TreatAsAtomicUnit=on
  Merge : Merge
  Min : MinMax  Inputs=2
  Multiport Switch1 : MultiPortSwitch  DataPortOrder=Zero-based contiguous  Inputs=11  zeroidx=on
  Multiport Switch2 : MultiPortSwitch  DataPortOrder=Zero-based contiguous  Inputs=11  zeroidx=on
  No Function 2 LCK : Lookup_n-D  NumberOfTableDimensions=1  BreakpointsForDimension1=P_LCS_VehicleSpd_TabX_Kph  Table=P_LCS_LATC_LCKAngleSlope_ratio  ExtrapMethod=Clip  InternalRulePriority=Speed  RndMeth=Simplest  InputSameDT=on
  Product : Product
  Switch Case : SwitchCase  CaseConditions={[1,2,3,4,5]}
  Switch Case Action Subsystem : Subsystem  TreatAsAtomicUnit=on
  Switch Case Action Subsystem1 : Subsystem  TreatAsAtomicUnit=on
  Unit Delay3 : UnitDelay  SampleTime=-1  HasFrameUpgradeWarning=on
  Unit Delay4 : UnitDelay  SampleTime=-1  HasFrameUpgradeWarning=on
  Unit Delay5 : UnitDelay  SampleTime=-1  HasFrameUpgradeWarning=on
  VehSpd_kph1 : InportShadow  Port=2
  Max_Lateral_Acc : Outport  OutDataTypeStr=single
  SteerAngSlope : Outport  Port=2  OutDataTypeStr=single
  wires:
  Data Type Conversion1/1 -> SteerAngSlope/1
  Data Type Conversion/1 -> Max_Lateral_Acc/1
  LCNomal_MaxAy/1 -> Multiport Switch2/5
  LKA_MaxAy/1 -> Multiport Switch2/6
  LCKMaxAy/1 -> Multiport Switch2/3
  LCKIEMaxAy/1 -> Multiport Switch2/4
  ELK_MaxAy/1 -> Multiport Switch2/7
  VehSpd_kph1/1 -> LCKMaxAy/1, LCNomal_MaxAy/1, LC_CancelMaxAy/1, LC_SportMaxAy/1, LC_Eco_MaxAy/1, ESS AES_MaxAy/1, ELK_MaxAy/1, LKA_MaxAy/1, LCKIEMaxAy/1
  ESS AES_MaxAy/1 -> Multiport Switch2/8
  LC_Eco_MaxAy/1 -> Multiport Switch2/9
  LC_SportMaxAy/1 -> Multiport Switch2/10
  LC_CancelMaxAy/1 -> Multiport Switch2/11
  Constant5/1 -> Multiport Switch2/12
  Constant1/1 -> Multiport Switch2/2
  Multiport Switch2/1 -> Data Type Conversion/1  "LCS_LATC_MaxAy_ms2"
  LC Cancel/1 -> Multiport Switch1/11
  LCK/IE TO LC_Sport/1 -> Multiport Switch1/10
  LCK/IE TO LC_Eco/1 -> Multiport Switch1/9
  ESS AES Active/1 -> Multiport Switch1/8
  Unit Delay5/1 -> MATLAB Function3/3(TarDangerLevelK1)
  VehSpd_kph/1 -> LCKIE_Active/1, LKA Active/1, ELK Active/1, ESS AES Active/1, LCK/IE TO LC_Eco/1, LCK/IE TO LC_Sport/1, LC Cancel/1, LCK/IE TO LC_Nomal/1, No Function 2 LCK/1
  ELK Active/1 -> Multiport Switch1/7
  LCKIE_Active/1 -> Multiport Switch1/4
  Unit Delay3/1 -> MATLAB Function3/5(CntK1)
  Unit Delay4/1 -> MATLAB Function3/4(FLgK1)
  Constant/1 -> Multiport Switch1/2
  MATLAB Function3/2(Cnt) -> Product/2, Unit Delay3/1
  MATLAB Function3/1(FLg) -> Switch Case/1, Switch Case Action Subsystem/1(Flg), Unit Delay4/1  "LCS_LATC_AngleSlopeFlg_st"
  Constant2/1 -> MATLAB Function3/1(delytime)
  Multiport Switch1/1 -> Min/2  "LCS_LATC_StateAngleSlope_degs"
  No Function 2 LCK/1 -> Multiport Switch1/3
  LKA Active/1 -> Multiport Switch1/6
  Constant4/1 -> Multiport Switch1/12
  Constant3/1 -> Product/1
  Product/1 -> [HoldTime]  "LCS_LATC_HoldTime_s"
  Min/1 -> Data Type Conversion1/1
  LCK/IE TO LC_Nomal/1 -> Multiport Switch1/5
  Switch Case/1 -> Switch Case Action Subsystem/Action
  Switch Case/2 -> Switch Case Action Subsystem1/Action
  [HoldTime] -> Switch Case Action Subsystem/2(StateHoldTime)
  Switch Case Action Subsystem/1(Out1) -> Merge/2
  Switch Case Action Subsystem1/1(Out1) -> Merge/1
  Merge/1 -> Min/1  "LCS_LATC_StateActAngleSlope_degs"
  TarDangerlLevel/1 -> MATLAB Function3/2(TarDangerLevel), Unit Delay5/1, Multiport Switch2/1, Multiport Switch1/1

== system PvtSubSys_LATC/LATC/LateralControl/LCS_Angle/Lateral_Control/kinematics_MPC/Understeer&Offset_Calc ==
  note: %% 匀速
  SteerAngle_deg : Inport
  PsiDtOpt : Inport  Port=2
  axvRef : Inport  Port=3
  vxvRef : Inport  Port=4
  DesLineC2 : Inport  Port=5
  Abs : Abs
  Abs2 : Abs
  Compare To Constant1 : simulink/Logic and Bit Operations/Compare To Constant  relop=>  const=P_LCS_LATC_CurOffsetVehicleSpdLimitValue_degs  OutDataTypeStr=boolean
  Compare To Constant6 : simulink/Logic and Bit Operations/Compare To Constant  relop=<=  const=1.5  OutDataTypeStr=boolean
  Constant1 : Constant  Value=P_Global_SteeringAngleRatio
  Constant2 : Constant  Value=P_LCS_LATC_CurOffsetA2FliterT_s  OutDataTypeStr=single
  Constant4 : Constant  Value=P_Global_CharSpd_ms
  Constant5 : Constant  Value=P_Global_WheelBase_m
  Constant6 : Constant  Value=57.3  OutDataTypeStr=single
  Enabled Subsystem : Subsystem  TreatAsAtomicUnit=on
  FilterTime2 : Product  Inputs=*//  RndMeth=Zero
  Gain : Gain  Gain=2
  LP filter : Subsystem
  Logical Operator : Logic  AllPortsSameDT=off  OutDataTypeStr=boolean
  Memory52 : Memory  InheritSampleTime=on
  Sum : Sum  Inputs=+-
  Terminator : Terminator
  YOD_Ackman : MATLAB Function  TreatAsAtomicUnit=on
  SteerAngleOffset_deg : Outport
  wires:
  Constant2/1 -> LP filter/2(TorqFilterTime)
  Gain/1 -> Abs/1
  Abs/1 -> LP filter/1(Raw)
  DesLineC2/1 -> Gain/1
  SteerAngle_deg/1 -> FilterTime2/1
  Compare To Constant1/1 -> Logical Operator/2
  YOD_Ackman/2(PsiDtAck) -> Memory52/1, Sum/1
  Enabled Subsystem/1(SteerAngleOffset_deg) -> SteerAngleOffset_deg/1
  Constant5/1 -> YOD_Ackman/3(WheelBase)
  Constant4/1 -> YOD_Ackman/2(Vch)
  Memory52/1 -> YOD_Ackman/5(PsiDtAckK1)
  PsiDtOpt/1 -> Sum/2
  vxvRef/1 -> YOD_Ackman/1(VxvRef), Compare To Constant1/1
  Sum/1 -> Enabled Subsystem/2(Raw)
  Logical Operator/1 -> Enabled Subsystem/Enable, Terminator/1  "LCS_OffSetUpdate_Flg"
  Constant1/1 -> FilterTime2/2
  Constant6/1 -> FilterTime2/3
  YOD_Ackman/1(AckConst) -> Enabled Subsystem/1(AckConst)
  FilterTime2/1 -> YOD_Ackman/4(AlpWheelAngle)
  axvRef/1 -> Abs2/1
  Abs2/1 -> Compare To Constant6/1
  Compare To Constant6/1 -> Logical Operator/1
  LP filter/1(output) -> Enabled Subsystem/3(Curve)

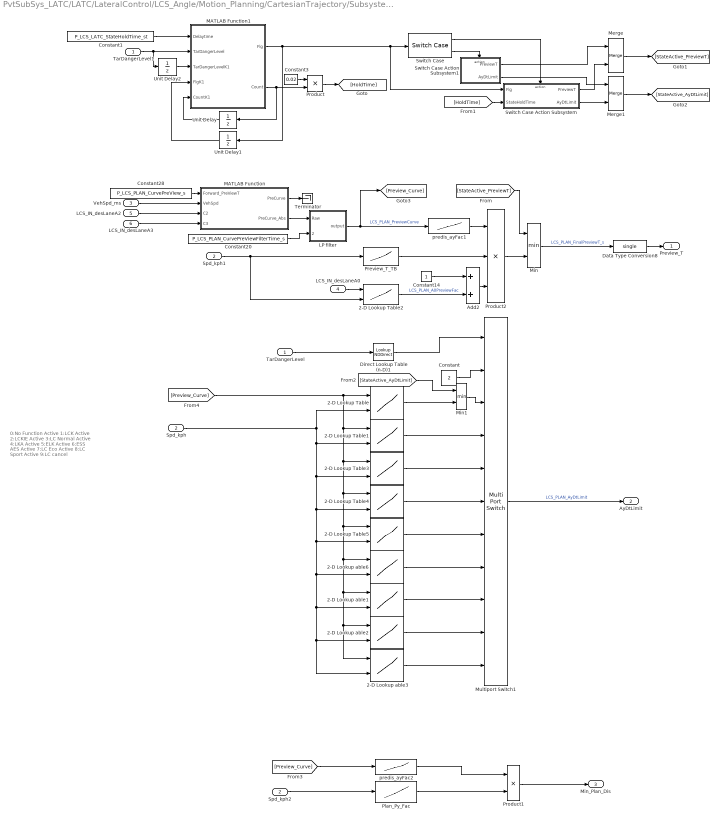
== system PvtSubSys_LATC/LATC/LateralControl/LCS_Angle/Motion_Planning/CartesianTrajectory/Subsystem1 ==
  note: 0:No Function Active
      | 1:LCK Active
      | 2:LCKIE Active
      | 3:LC Normal Active
      | 4:LKA Active
      | 5:ELK Active
      | 6:ESS AES Active
      | 7:LC Eco Active
      | 8:LC Sport Active
      | 9:LC cancel
  TarDangerLevel : Inport
  Spd_kph : Inport  Port=2
  VehSpd_ms : Inport  Port=3
  LCS_IN_desLaneA0 : Inport  Port=4
  LCS_IN_desLaneA2 : Inport  Port=5
  LCS_IN_desLaneA3 : Inport  Port=6
  2-D Lookup Table : Lookup_n-D  BreakpointsForDimension1=P_LCS_PLAN_PreDisCurve_TabX_m  BreakpointsForDimension2=P_LCS_PLAN_VehicleSpd_TabY_Kph  Table=P_LCS_PLAN_LCKAyDtLimit_Tab_ms3  InternalRulePriority=Speed  RndMeth=Simplest  InputSameDT=on
      settings: InputPortMap=u0,u1
  2-D Lookup Table1 : Lookup_n-D  BreakpointsForDimension1=P_LCS_PLAN_PreDisCurve_TabX_m  BreakpointsForDimension2=P_LCS_PLAN_VehicleSpd_TabY_Kph  Table=P_LCS_PLAN_LCKIEAyDtLimit_Tab_ms3  InternalRulePriority=Speed  RndMeth=Simplest  InputSameDT=on
      settings: InputPortMap=u0,u1
  2-D Lookup Table2 : Lookup_n-D  BreakpointsForDimension1=P_LCS_PLAN_A0Distance_TabX_m  BreakpointsForDimension2=P_LCS_PLAN_VehicleSpd_TabX_kph  Table=P_LCS_PLAN_A0PreViewFac_ratio  ExtrapMethod=Clip  UseLastTableValue=on  InternalRulePriority=Speed  RndMeth=Simplest  InputSameDT=on
      settings: InputPortMap=u0,u1
  2-D Lookup Table3 : Lookup_n-D  BreakpointsForDimension1=P_LCS_PLAN_PreDisCurve_TabX_m  BreakpointsForDimension2=P_LCS_PLAN_VehicleSpd_TabY_Kph  Table=P_LCS_PLAN_LCNormalAyDtLimit_Tab_ms3  InternalRulePriority=Speed  RndMeth=Simplest  InputSameDT=on
      settings: InputPortMap=u0,u1
  2-D Lookup Table4 : Lookup_n-D  BreakpointsForDimension1=P_LCS_PLAN_PreDisCurve_TabX_m  BreakpointsForDimension2=P_LCS_PLAN_VehicleSpd_TabY_Kph  Table=P_LCS_PLAN_LKAAyDtLimit_Tab_ms3  InternalRulePriority=Speed  RndMeth=Simplest  InputSameDT=on
      settings: InputPortMap=u0,u1
  2-D Lookup Table5 : Lookup_n-D  BreakpointsForDimension1=P_LCS_PLAN_PreDisCurve_TabX_m  BreakpointsForDimension2=P_LCS_PLAN_VehicleSpd_TabY_Kph  Table=P_LCS_PLAN_ELKAyDtLimit_Tab_ms3  InternalRulePriority=Speed  RndMeth=Simplest  InputSameDT=on
      settings: InputPortMap=u0,u1
  2-D Lookup able1 : Lookup_n-D  BreakpointsForDimension1=P_LCS_PLAN_PreDisCurve_TabX_m  BreakpointsForDimension2=P_LCS_PLAN_VehicleSpd_TabY_Kph  Table=P_LCS_PLAN_LCEcoAyDtLimit_Tab_ms3  InternalRulePriority=Speed  RndMeth=Simplest  InputSameDT=on
      settings: InputPortMap=u0,u1
  2-D Lookup able2 : Lookup_n-D  BreakpointsForDimension1=P_LCS_PLAN_PreDisCurve_TabX_m  BreakpointsForDimension2=P_LCS_PLAN_VehicleSpd_TabY_Kph  Table=P_LCS_PLAN_LCSportAyDtLimit_Tab_ms3  InternalRulePriority=Speed  RndMeth=Simplest  InputSameDT=on
      settings: InputPortMap=u0,u1
  2-D Lookup able3 : Lookup_n-D  BreakpointsForDimension1=P_LCS_PLAN_PreDisCurve_TabX_m  BreakpointsForDimension2=P_LCS_PLAN_VehicleSpd_TabY_Kph  Table=P_LCS_PLAN_LCCancleAyDtLimit_Tab_ms3  InternalRulePriority=Speed  RndMeth=Simplest  InputSameDT=on
      settings: InputPortMap=u0,u1
  2-D Lookup able6 : Lookup_n-D  BreakpointsForDimension1=P_LCS_PLAN_PreDisCurve_TabX_m  BreakpointsForDimension2=P_LCS_PLAN_VehicleSpd_TabY_Kph  Table=P_LCS_PLAN_ESSAyDtLimit_Tab_ms3  InternalRulePriority=Speed  RndMeth=Simplest  InputSameDT=on
      settings: InputPortMap=u0,u1
  Add2 : Sum
  Constant : Constant  Value=2  OutDataTypeStr=single
  Constant1 : Constant  Value=P_LCS_LATC_StateHoldTime_st  OutDataTypeStr=uint16
  Constant14 : Constant  OutDataTypeStr=single
  Constant20 : Constant  Value=P_LCS_PLAN_CurvePreViewFilterTime_s
  Constant28 : Constant  Value=P_LCS_PLAN_CurvePreView_s  OutDataTypeStr=single
  Constant3 : Constant  Value=0.02
  Data Type Conversion8 : DataTypeConversion  OutDataTypeStr=single
  Direct Lookup Table (n-D)1 : LookupNDDirect  NumberOfTableDimensions=1  Table=[0 1 2 3 4 5 6 7 8 9]  TableDataTypeStr=uint8
  LP filter : Subsystem
  MATLAB Function : MATLAB Function  TreatAsAtomicUnit=on
  MATLAB Function1 : MATLAB Function  TreatAsAtomicUnit=on
  Merge : Merge
  Merge1 : Merge
  Min : MinMax  Inputs=2
  Min1 : MinMax  Inputs=2
  Multiport Switch1 : MultiPortSwitch  DataPortOrder=Zero-based contiguous  Inputs=10  zeroidx=on
  Plan_Py_Fac : Lookup_n-D  NumberOfTableDimensions=1  BreakpointsForDimension1=P_LCS_PLAN_VehicleSpd_TabX_kph  Table=P_LCS_PLAN_MinPlanDis_m  ExtrapMethod=Clip  UseLastTableValue=on  InternalRulePriority=Speed  RndMeth=Simplest  InputSameDT=on
  Preview_T_TB : Lookup_n-D  NumberOfTableDimensions=1  BreakpointsForDimension1=P_LCS_PLAN_VehicleSpd_TabX_kph  Table=P_LCS_PLAN_PreViewT_Tab_s  ExtrapMethod=Clip  UseLastTableValue=on  InternalRulePriority=Speed  RndMeth=Simplest  InputSameDT=on
  Product : Product
  Product1 : Product
  Product2 : Product  Inputs=3
  Spd_kph1 : InportShadow  Port=2
  Spd_kph2 : InportShadow  Port=2
  Switch Case : SwitchCase  CaseConditions={[1]}
  Switch Case Action Subsystem : Subsystem  TreatAsAtomicUnit=on
  Switch Case Action Subsystem1 : Subsystem  TreatAsAtomicUnit=on
  TarDangerLevel1 : InportShadow
  Terminator : Terminator
  Unit Delay : UnitDelay  SampleTime=-1  HasFrameUpgradeWarning=on
  Unit Delay1 : UnitDelay  SampleTime=-1  HasFrameUpgradeWarning=on
  Unit Delay2 : UnitDelay  SampleTime=-1  HasFrameUpgradeWarning=on
  predis_ayFac1 : Lookup_n-D  NumberOfTableDimensions=1  BreakpointsForDimension1=P_LCS_PLAN_CurvePreview_TabX_m  Table=P_LCS_PLAN_CurvePreview_Tab_ratio  ExtrapMethod=Clip  UseLastTableValue=on  InternalRulePriority=Speed  RndMeth=Simplest  InputSameDT=on
  predis_ayFac2 : Lookup_n-D  NumberOfTableDimensions=1  BreakpointsForDimension1=P_LCS_PLAN_CurvePreview_TabX_m  Table=P_LCS_PLAN_PreCurMinDisFac_ratio  ExtrapMethod=Clip  UseLastTableValue=on  InternalRulePriority=Speed  RndMeth=Simplest  InputSameDT=on
  Preview_T : Outport  OutDataTypeStr=single
  AyDtLimit : Outport  Port=2  OutDataTypeStr=single
  Min_Plan_Dis : Outport  Port=3  OutDataTypeStr=single
  wires:
  2-D Lookup able3/1 -> Multiport Switch1/11
  2-D Lookup able2/1 -> Multiport Switch1/10
  2-D Lookup able1/1 -> Multiport Switch1/9
  2-D Lookup able6/1 -> Multiport Switch1/8
  2-D Lookup Table4/1 -> Multiport Switch1/6
  Spd_kph/1 -> 2-D Lookup Table5/2, 2-D Lookup able6/2, 2-D Lookup able1/2, 2-D Lookup able2/2, 2-D Lookup able3/2, 2-D Lookup Table4/2, 2-D Lookup Table3/2, 2-D Lookup Table1/2, 2-D Lookup Table/2
  [Preview_Curve] -> 2-D Lookup Table/1, 2-D Lookup Table1/1, 2-D Lookup Table3/1, 2-D Lookup Table4/1, 2-D Lookup Table5/1, 2-D Lookup able6/1, 2-D Lookup able1/1, 2-D Lookup able2/1, 2-D Lookup able3/1
  MATLAB Function/1(PreCurve) -> Terminator/1
  MATLAB Function/2(PreCurve_Abs) -> LP filter/1(Raw)
  predis_ayFac2/1 -> Product1/1
  Product1/1 -> Min_Plan_Dis/1
  [Preview_Curve] -> predis_ayFac2/1
  Spd_kph2/1 -> Plan_Py_Fac/1
  Plan_Py_Fac/1 -> Product1/2
  Direct Lookup Table (n-D)1/1 -> Multiport Switch1/1
  TarDangerLevel/1 -> Direct Lookup Table (n-D)1/1
  Multiport Switch1/1 -> AyDtLimit/1  "LCS_PLAN_AyDtLimit"
  2-D Lookup Table/1 -> Min1/2
  Preview_T_TB/1 -> Product2/2
  2-D Lookup Table2/1 -> Add2/2  "LCS_PLAN_A0PreviewFac"
  Constant14/1 -> Add2/1
  Add2/1 -> Product2/3
  Spd_kph1/1 -> 2-D Lookup Table2/2, Preview_T_TB/1
  LCS_IN_desLaneA0/1 -> 2-D Lookup Table2/1
  Min/1 -> Data Type Conversion8/1  "LCS_PLAN_FinalPreviewT_s"
  Data Type Conversion8/1 -> Preview_T/1
  VehSpd_ms/1 -> MATLAB Function/2(VehSpd)
  LCS_IN_desLaneA2/1 -> MATLAB Function/3(C2)
  LCS_IN_desLaneA3/1 -> MATLAB Function/4(C3)
  Constant20/1 -> LP filter/2(TorqFilterTime)
  LP filter/1(output) -> predis_ayFac1/1, [Preview_Curve]  "LCS_PLAN_PreviewCurve"
  predis_ayFac1/1 -> Product2/1
  Constant28/1 -> MATLAB Function/1(Forward_PreViewT)
  Constant/1 -> Multiport Switch1/2
  2-D Lookup Table1/1 -> Multiport Switch1/4
  2-D Lookup Table3/1 -> Multiport Switch1/5
  2-D Lookup Table5/1 -> Multiport Switch1/7
  Unit Delay/1 -> MATLAB Function1/5(CountK1)
  Unit Delay1/1 -> MATLAB Function1/4(FlgK1)
  TarDangerLevel1/1 -> Unit Delay2/1, MATLAB Function1/2(TarDangerLevel)
  Unit Delay2/1 -> MATLAB Function1/3(TarDangerLevelK1)
  Constant1/1 -> MATLAB Function1/1(Delaytime)
  MATLAB Function1/1(Flg) -> Unit Delay1/1, Switch Case Action Subsystem/1(Flg), Switch Case/1
  Switch Case Action Subsystem1/1(PreviewT) -> Merge/1
  Switch Case/1 -> Switch Case Action Subsystem/Action
  Switch Case Action Subsystem/1(PreviewT) -> Merge/2
  MATLAB Function1/2(Count) -> Product/2, Unit Delay/1
  Switch Case/2 -> Switch Case Action Subsystem1/Action
  Constant3/1 -> Product/1
  [HoldTime] -> Switch Case Action Subsystem/2(StateHoldTime)
  Product/1 -> [HoldTime]
  Switch Case Action Subsystem/2(AyDtLimit) -> Merge1/2
  Switch Case Action Subsystem1/2(AyDtLimit) -> Merge1/1
  Merge/1 -> [StateActive_PreviewT]
  Merge1/1 -> [StateActive_AyDtLimit]
  [StateActive_PreviewT] -> Min/1
  Product2/1 -> Min/2
  [StateActive_AyDtLimit] -> Min1/1
  Min1/1 -> Multiport Switch1/3
